simulink model "lab"  (R2022b)
settings: Solver=ode23tb  StartTime=0.0  StopTime=100e-3  MaxStep=10e-6  RelTol=1e-3
libraries: spsACVoltageSourceLib x2, spsMonostableLib x2, spsRMSLib x2, spsThyristorLib x2, spsVoltageMeasurementLib x2, spsCurrentMeasurementLib x1, spsDiodeLib x1, spsSeriesRLCBranchLib x1, sps_lib x1
settings Model: Creator=Student  LastModifiedBy=Student

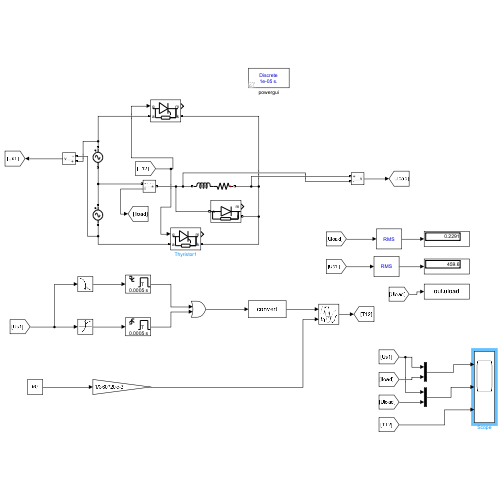
[thumbnail: Simulink's stored preview of the top-level diagram]
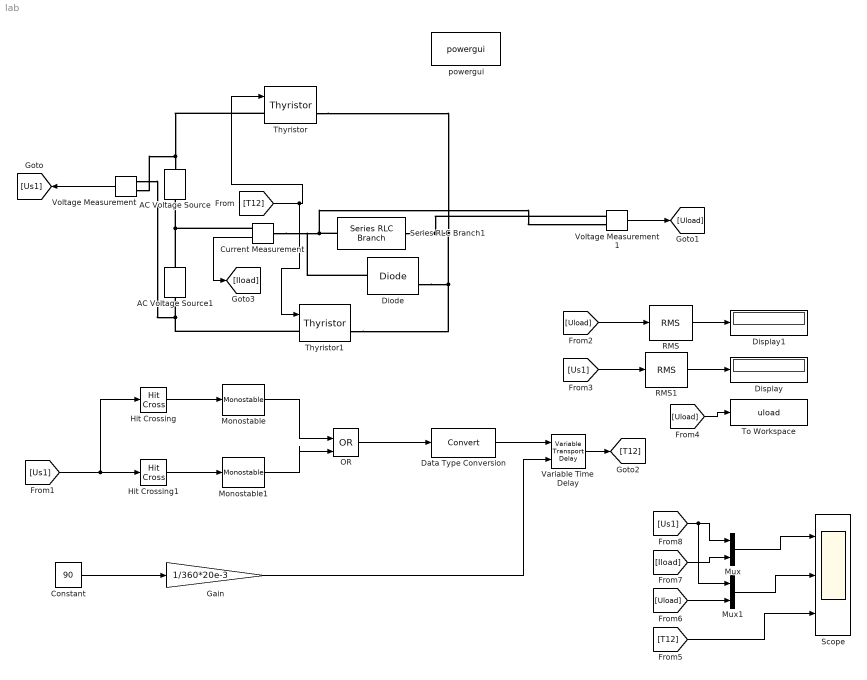
== system lab ==
  AC Voltage Source : spsACVoltageSourceLib/AC Voltage Source  Amplitude=325  Phase=0  Frequency=50  SampleTime=0  Measurements=Voltage  BusType=swing  Pref=10e3  Qref=0  Qmin=-inf  Qmax=+inf
  AC Voltage Source1 : spsACVoltageSourceLib/AC Voltage Source  Amplitude=325  Phase=0  Frequency=50  SampleTime=0  Measurements=Voltage  BusType=swing  Pref=10e3  Qref=0  Qmin=-inf  Qmax=+inf
  Constant : Constant  Value=90
  Current Measurement : spsCurrentMeasurementLib/Current Measurement  PhasorSimulation=off  OutputType=Complex  PSBequivalent=0
  Data Type Conversion : DataTypeConversion  SaturateOnIntegerOverflow=off  RndMeth=Floor
  Diode : spsDiodeLib/Diode  Ron=0.001  Lon=0  Vf=0.8  IC=0  UseSnubber=0  Rs=500  Cs=250e-9  Measurements=on
  Display : Display
  Display1 : Display
  Gain : Gain  Gain=1/360*20e-3
  Hit Crossing : HitCross  HitCrossingDirection=falling
  Hit Crossing1 : HitCross  HitCrossingDirection=rising
  Monostable : spsMonostableLib/Monostable  EdgeDetect=Falling  PulseDuration=0.0005  ic=0  Ts=0
      settings: LibrarySourceBlock=sps_lib/Control/Monostable
  Monostable1 : spsMonostableLib/Monostable  EdgeDetect=Rising  PulseDuration=0.0005  ic=0  Ts=0
      settings: LibrarySourceBlock=sps_lib/Control/Monostable
  Mux : Mux  Inputs=2
  Mux1 : Mux  Inputs=2
  OR : Logic  Operator=OR  IconShape=distinctive  AllPortsSameDT=off  OutDataTypeStr=boolean
  RMS : spsRMSLib/RMS  TrueRMS=off  Freq=50  RMSInit=0  Ts=0
  RMS1 : spsRMSLib/RMS  TrueRMS=off  Freq=50  RMSInit=0  Ts=0
  Scope : Scope  NumInputPorts=3
  Series RLC Branch1 : spsSeriesRLCBranchLib/Series RLC Branch  LConnTagsString=__new0  RConnTagsString=__new0  BranchType=RL  Resistance=2  Inductance=1e-3  SetiL0=off  InitialCurrent=0  Capacitance=1e-6  Setx0=off  InitialVoltage=0  Measurements=None
  Thyristor : spsThyristorLib/Thyristor  Ron=0.001  Lon=0  Vf=0.8  IC=0  Rs=500  Cs=250e-9  Measurements=on
  Thyristor1 : spsThyristorLib/Thyristor  Ron=0.001  Lon=0  Vf=0.8  IC=0  Rs=500  Cs=250e-9  Measurements=on
  To Workspace : ToWorkspace  VariableName=uload  SaveFormat=Timeseries  SampleTime=-1
  Variable Time Delay : VariableTransportDelay  MaximumDelay=10
  Voltage Measurement : spsVoltageMeasurementLib/Voltage Measurement  PhasorSimulation=off  OutputType=Complex  PSBequivalent=0
  Voltage Measurement1 : spsVoltageMeasurementLib/Voltage Measurement  PhasorSimulation=off  OutputType=Complex  PSBequivalent=0
  powergui : sps_lib/powergui  Priority=1  SimulationMode=Discrete  SampleTime=1e-05  frequency=60  Iterations=50  frequencyindice=50  Pbase=100e6  ErrMax=1e-4  UnitsV=kV  UnitsW=MW  buscounter=0  FunctionMessages=off  echomessages=off  EnableUseOfTLC=off  CurrentSourceSwitches=off  DisableSnubberDevices=off  DisableRonSwitches=off  DisableVfSwitches=off  DisplayEquations=off  AutomaticDiscreteSolvers=off  SolverType=Tustin/Backward Euler (TBE)  Interpol=off  ExternalGateDelay=off  methode=off  Ts=100  x0status=blocks  SPID=on  SwTol=0  HookPort=off  NonlinearTolerance=1e-4  nMaxIteration=100  ContinueOnMaxIteration=off  RestoreLinks=warning  ResistiveCurrentMeasurement=off  Frange=[0:2:500]  Ylog=off  Xlog=on  ShowGrid=off  save=off  variable=ZData  structure=0  ZoomFFT=off  StartTime=0.0  cycles=1  DisplayStyle=1  fundamental=60  FreqAxis=off  MaxFrequency=1000  frequencyindicesteady=1  RmsSteady=1  display=off
  wires:
  Voltage Measurement/1 -> [Us1]
  [T12] -> Thyristor1/1, Thyristor/1
  Voltage Measurement1/1 -> [Uload]
  [Us1] -> Hit Crossing/1, Hit Crossing1/1
  Hit Crossing/1 -> Monostable/1
  Hit Crossing1/1 -> Monostable1/1
  Monostable/1 -> OR/1
  Monostable1/1 -> OR/2
  OR/1 -> Data Type Conversion/1
  Data Type Conversion/1 -> Variable Time Delay/1
  Constant/1 -> Gain/1
  Gain/1 -> Variable Time Delay/2
  Variable Time Delay/1 -> [T12]
  RMS1/1 -> Display/1
  RMS/1 -> Display1/1
  [Uload] -> RMS/1
  [Us1] -> RMS1/1
  [Uload] -> To Workspace/1
  Mux/1 -> Scope/1
  Mux1/1 -> Scope/2
  [T12] -> Scope/3
  [Uload] -> Mux1/2
  Current Measurement/1 -> [Iload]
  [Us1] -> Mux1/1, Mux/1
  [Iload] -> Mux/2
  connections:
  AC Voltage Source/RConn1 -- Thyristor/LConn1 -- Voltage Measurement/LConn1
  Thyristor1/LConn1 -- Voltage Measurement/LConn2 -- AC Voltage Source1/LConn1
  AC Voltage Source1/RConn1 -- Current Measurement/RConn1 -- AC Voltage Source/LConn1
  Thyristor1/RConn1 -- Diode/RConn1 -- Thyristor/RConn1 -- Voltage Measurement1/LConn1 -- Series RLC Branch1/LConn1
  Series RLC Branch1/RConn1 -- Diode/LConn1 -- Current Measurement/LConn1 -- Voltage Measurement1/LConn2
